simulink model "Comparison_to_Nest"  (R2020b)
settings: Solver=VariableStepAuto  StartTime=0.0  StopTime=0.4  RelTol=1e-3
libraries: NeuroModelerLibrary x7
settings Model: Creator=Александра  LastModifiedBy=Александра

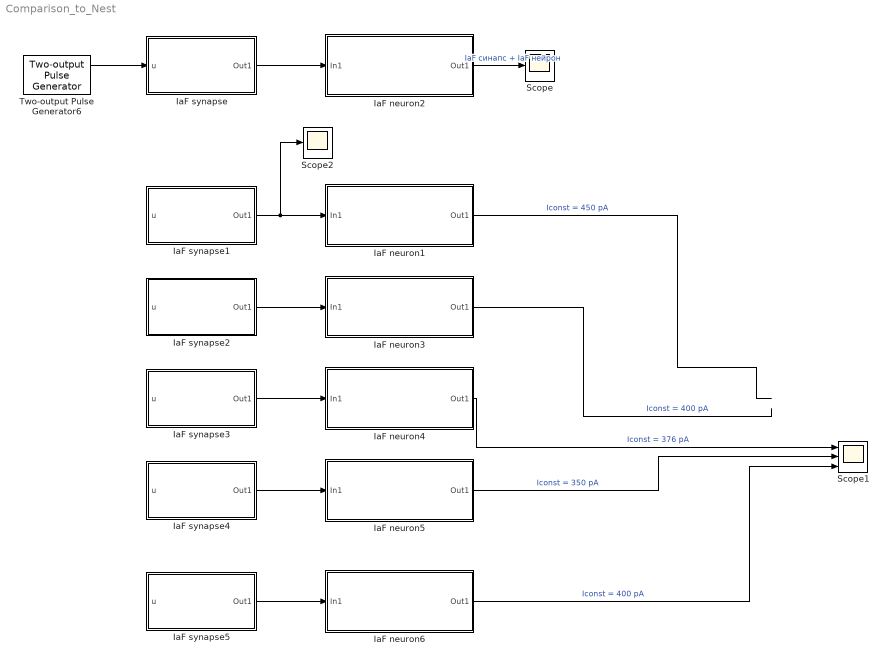
== system Comparison_to_Nest ==
  IaF neuron1 : Subsystem  mask{tau_m=0.010, Cm=250e-12, I_const=450e-12, E_L=-0.070, V_reset=-0.070, V_th=-0.055}
      mask prompts: tau_m "Membrane time constatnt"; Cm "Membrane capacity"; I_const "Constant input current"; E_L "Resting membrane potential"; V_reset "Reset membrane potential"; V_th "Threshold potential"
  IaF neuron2 : Subsystem  mask{tau_m=0.01, Cm=250e-12, I_const=0, E_L=-0.070, V_reset=-0.10, V_th=-0.055}
      mask prompts: tau_m "Membrane time constatnt"; Cm "Membrane capacity"; I_const "Constant input current"; E_L "Resting membrane potential"; V_reset "Reset membrane potential"; V_th "Threshold potential"
  IaF neuron3 : Subsystem  mask{tau_m=0.010, Cm=250e-12, I_const=400e-12, E_L=-0.070, V_reset=-0.070, V_th=-0.055}
      mask prompts: tau_m "Membrane time constatnt"; Cm "Membrane capacity"; I_const "Constant input current"; E_L "Resting membrane potential"; V_reset "Reset membrane potential"; V_th "Threshold potential"
  IaF neuron4 : Subsystem  mask{tau_m=0.010, Cm=250e-12, I_const=376e-12, E_L=-0.070, V_reset=-0.070, V_th=-0.055}
      mask prompts: tau_m "Membrane time constatnt"; Cm "Membrane capacity"; I_const "Constant input current"; E_L "Resting membrane potential"; V_reset "Reset membrane potential"; V_th "Threshold potential"
  IaF neuron5 : Subsystem  mask{tau_m=0.010, Cm=250e-12, I_const=350e-12, E_L=-0.070, V_reset=-0.070, V_th=-0.055}
      mask prompts: tau_m "Membrane time constatnt"; Cm "Membrane capacity"; I_const "Constant input current"; E_L "Resting membrane potential"; V_reset "Reset membrane potential"; V_th "Threshold potential"
  IaF neuron6 : Subsystem  mask{tau_m=0.010, Cm=250e-12, I_const=400e-12, E_L=-0.070, V_reset=-0.070, V_th=-0.055}
      mask prompts: tau_m "Membrane time constatnt"; Cm "Membrane capacity"; I_const "Constant input current"; E_L "Resting membrane potential"; V_reset "Reset membrane potential"; V_th "Threshold potential"
  IaF synapse : Subsystem  mask{tau_syn=2e-3, I_syn=1e-8, weight=1, delay=1e-3}
      mask prompts: tau_syn "Rise time of the excitatory synaptic alpha function"; I_syn "Synaptic current amplitude"
  IaF synapse1 : Subsystem  mask{tau_syn=2e-3, I_syn=1e-8, weight=1, delay=1e-3}
      mask prompts: tau_syn "Rise time of the excitatory synaptic alpha function"; I_syn "Synaptic current amplitude"
  IaF synapse2 : Subsystem  mask{tau_syn=2e-3, I_syn=1e-8, weight=1, delay=1e-3}
      mask prompts: tau_syn "Rise time of the excitatory synaptic alpha function"; I_syn "Synaptic current amplitude"
  IaF synapse3 : Subsystem  mask{tau_syn=2e-3, I_syn=1e-8, weight=1, delay=1e-3}
      mask prompts: tau_syn "Rise time of the excitatory synaptic alpha function"; I_syn "Synaptic current amplitude"
  IaF synapse4 : Subsystem  mask{tau_syn=2e-3, I_syn=1e-8, weight=1, delay=1e-3}
      mask prompts: tau_syn "Rise time of the excitatory synaptic alpha function"; I_syn "Synaptic current amplitude"
  IaF synapse5 : Subsystem  mask{tau_syn=2e-3, I_syn=1e-8, weight=1, delay=1e-3}
      mask prompts: tau_syn "Rise time of the excitatory synaptic alpha function"; I_syn "Synaptic current amplitude"
  Scope : Scope
  Scope1 : Scope  NumInputPorts=3
  Scope2 : Scope
  Two-output Pulse Generator6 : NeuroModelerLibrary/Support/Two-output Pulse Generator  A=1  P1=200  P2=200  PW=1  ST=0.001  OOn1=0.1  OOff1=1.0  OOn2=0.1  OOff2=0.2
  wires:
  Two-output Pulse Generator6/1 -> IaF synapse/1(u)
  IaF synapse/1(Out1) -> IaF neuron2/1(In1)
  IaF neuron2/1(Out1) -> Scope/1  "IaF синапс + IaF нейрон"
  IaF neuron1/1(Out1) -> ?  "Iconst = 450 pA"
  IaF synapse1/1(Out1) -> Scope2/1, IaF neuron1/1(In1)
  IaF neuron3/1(Out1) -> ?  "Iconst = 400 pA"
  IaF synapse2/1(Out1) -> IaF neuron3/1(In1)
  IaF neuron4/1(Out1) -> Scope1/1  "Iconst = 376 pA"
  IaF synapse3/1(Out1) -> IaF neuron4/1(In1)
  IaF synapse4/1(Out1) -> IaF neuron5/1(In1)
  IaF synapse5/1(Out1) -> IaF neuron6/1(In1)
  IaF neuron5/1(Out1) -> Scope1/2  "Iconst = 350 pA"
  IaF neuron6/1(Out1) -> Scope1/3  "Iconst = 400 pA"

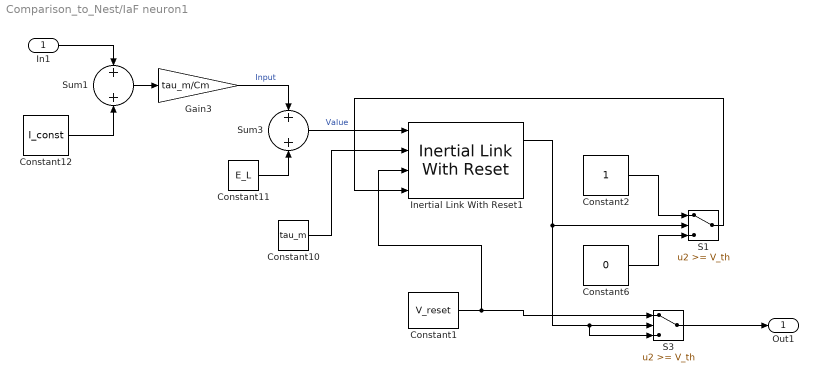
== system Comparison_to_Nest/IaF neuron1 ==
  In1 : Inport
  Constant1 : Constant  Value=V_reset
  Constant10 : Constant  Value=tau_m
  Constant11 : Constant  Value=E_L
  Constant12 : Constant  Value=I_const
  Constant2 : Constant
  Constant6 : Constant  Value=0
  Gain3 : Gain  Gain=tau_m/Cm
  Inertial Link With Reset1 : NeuroModelerLibrary/Support/Inertial Link With Reset  SystemSampleTime=-1  VariantActivationTime=update diagram  Latency=0  AutoFrameSizeCalculation=off
  S1 : Switch  Threshold=V_th  SaturateOnIntegerOverflow=on  InputSameDT=on
  S3 : Switch  Threshold=V_th  SaturateOnIntegerOverflow=on  InputSameDT=on
  Sum1 : Sum
  Sum3 : Sum
  Out1 : Outport
  wires:
  Constant11/1 -> Sum3/2
  Constant10/1 -> Inertial Link With Reset1/2
  In1/1 -> Sum1/1
  Sum1/1 -> Gain3/1
  Constant12/1 -> Sum1/2
  Constant2/1 -> S1/1
  Constant6/1 -> S1/3
  Sum3/1 -> Inertial Link With Reset1/1  "Value"
  Inertial Link With Reset1/1 -> S1/2, S3/3, S3/2
  Constant1/1 -> Inertial Link With Reset1/3, S3/1
  S1/1 -> Inertial Link With Reset1/4
  S3/1 -> Out1/1
  Gain3/1 -> Sum3/1  "Input"

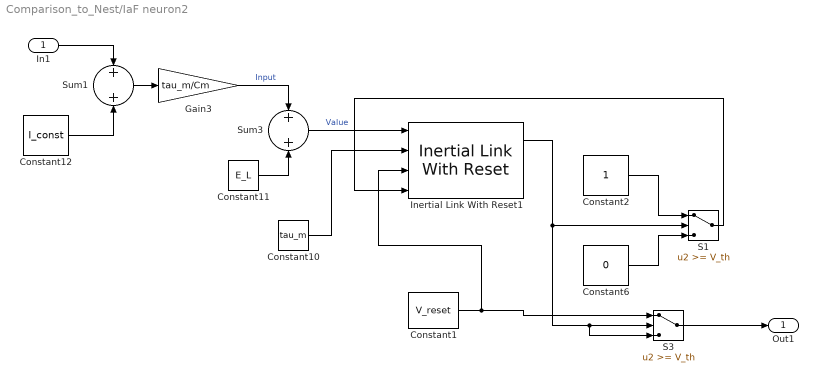
== system Comparison_to_Nest/IaF neuron2 ==
  In1 : Inport
  Constant1 : Constant  Value=V_reset
  Constant10 : Constant  Value=tau_m
  Constant11 : Constant  Value=E_L
  Constant12 : Constant  Value=I_const
  Constant2 : Constant
  Constant6 : Constant  Value=0
  Gain3 : Gain  Gain=tau_m/Cm
  Inertial Link With Reset1 : NeuroModelerLibrary/Support/Inertial Link With Reset  SystemSampleTime=-1  VariantActivationTime=update diagram  Latency=0  AutoFrameSizeCalculation=off
  S1 : Switch  Threshold=V_th  SaturateOnIntegerOverflow=on  InputSameDT=on
  S3 : Switch  Threshold=V_th  SaturateOnIntegerOverflow=on  InputSameDT=on
  Sum1 : Sum
  Sum3 : Sum
  Out1 : Outport
  wires:
  Constant11/1 -> Sum3/2
  Constant10/1 -> Inertial Link With Reset1/2
  In1/1 -> Sum1/1
  Sum1/1 -> Gain3/1
  Constant12/1 -> Sum1/2
  Constant2/1 -> S1/1
  Constant6/1 -> S1/3
  Sum3/1 -> Inertial Link With Reset1/1  "Value"
  Inertial Link With Reset1/1 -> S1/2, S3/3, S3/2
  Constant1/1 -> Inertial Link With Reset1/3, S3/1
  S1/1 -> Inertial Link With Reset1/4
  S3/1 -> Out1/1
  Gain3/1 -> Sum3/1  "Input"

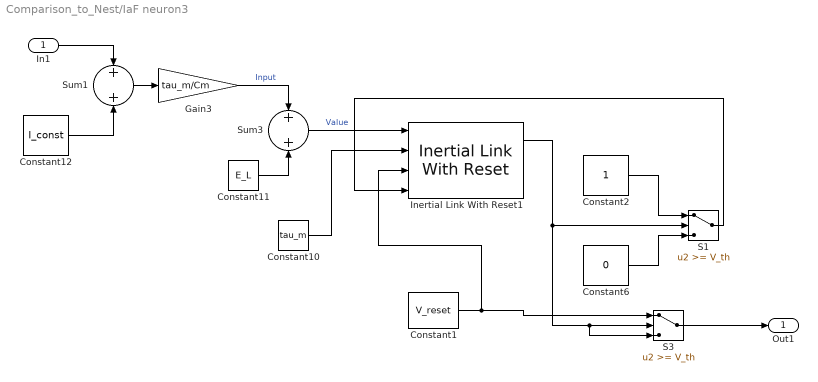
== system Comparison_to_Nest/IaF neuron3 ==
  In1 : Inport
  Constant1 : Constant  Value=V_reset
  Constant10 : Constant  Value=tau_m
  Constant11 : Constant  Value=E_L
  Constant12 : Constant  Value=I_const
  Constant2 : Constant
  Constant6 : Constant  Value=0
  Gain3 : Gain  Gain=tau_m/Cm
  Inertial Link With Reset1 : NeuroModelerLibrary/Support/Inertial Link With Reset  SystemSampleTime=-1  VariantActivationTime=update diagram  Latency=0  AutoFrameSizeCalculation=off
  S1 : Switch  Threshold=V_th  SaturateOnIntegerOverflow=on  InputSameDT=on
  S3 : Switch  Threshold=V_th  SaturateOnIntegerOverflow=on  InputSameDT=on
  Sum1 : Sum
  Sum3 : Sum
  Out1 : Outport
  wires:
  Constant11/1 -> Sum3/2
  Constant10/1 -> Inertial Link With Reset1/2
  In1/1 -> Sum1/1
  Sum1/1 -> Gain3/1
  Constant12/1 -> Sum1/2
  Constant2/1 -> S1/1
  Constant6/1 -> S1/3
  Sum3/1 -> Inertial Link With Reset1/1  "Value"
  Inertial Link With Reset1/1 -> S1/2, S3/3, S3/2
  Constant1/1 -> Inertial Link With Reset1/3, S3/1
  S1/1 -> Inertial Link With Reset1/4
  S3/1 -> Out1/1
  Gain3/1 -> Sum3/1  "Input"

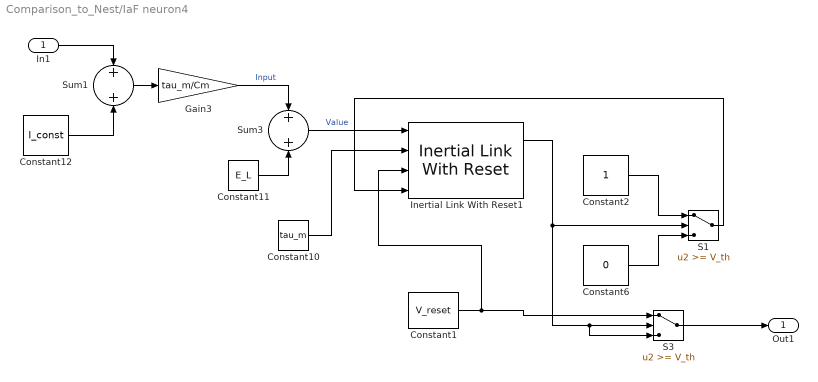
== system Comparison_to_Nest/IaF neuron4 ==
  In1 : Inport
  Constant1 : Constant  Value=V_reset
  Constant10 : Constant  Value=tau_m
  Constant11 : Constant  Value=E_L
  Constant12 : Constant  Value=I_const
  Constant2 : Constant
  Constant6 : Constant  Value=0
  Gain3 : Gain  Gain=tau_m/Cm
  Inertial Link With Reset1 : NeuroModelerLibrary/Support/Inertial Link With Reset  SystemSampleTime=-1  VariantActivationTime=update diagram  Latency=0  AutoFrameSizeCalculation=off
  S1 : Switch  Threshold=V_th  SaturateOnIntegerOverflow=on  InputSameDT=on
  S3 : Switch  Threshold=V_th  SaturateOnIntegerOverflow=on  InputSameDT=on
  Sum1 : Sum
  Sum3 : Sum
  Out1 : Outport
  wires:
  Constant11/1 -> Sum3/2
  Constant10/1 -> Inertial Link With Reset1/2
  In1/1 -> Sum1/1
  Sum1/1 -> Gain3/1
  Constant12/1 -> Sum1/2
  Constant2/1 -> S1/1
  Constant6/1 -> S1/3
  Sum3/1 -> Inertial Link With Reset1/1  "Value"
  Inertial Link With Reset1/1 -> S1/2, S3/3, S3/2
  Constant1/1 -> Inertial Link With Reset1/3, S3/1
  S1/1 -> Inertial Link With Reset1/4
  S3/1 -> Out1/1
  Gain3/1 -> Sum3/1  "Input"

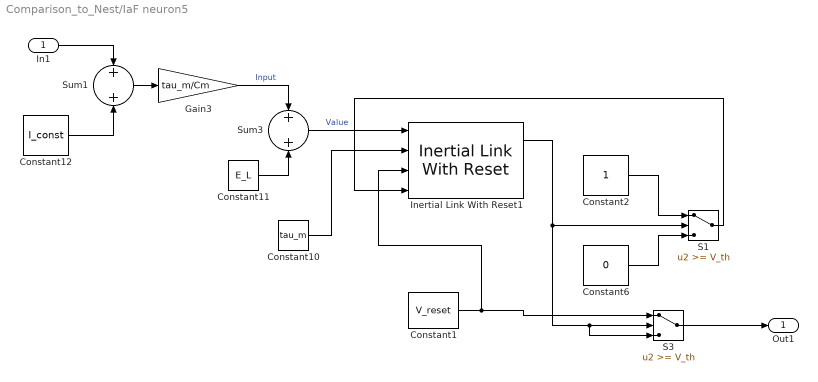
== system Comparison_to_Nest/IaF neuron5 ==
  In1 : Inport
  Constant1 : Constant  Value=V_reset
  Constant10 : Constant  Value=tau_m
  Constant11 : Constant  Value=E_L
  Constant12 : Constant  Value=I_const
  Constant2 : Constant
  Constant6 : Constant  Value=0
  Gain3 : Gain  Gain=tau_m/Cm
  Inertial Link With Reset1 : NeuroModelerLibrary/Support/Inertial Link With Reset  SystemSampleTime=-1  VariantActivationTime=update diagram  Latency=0  AutoFrameSizeCalculation=off
  S1 : Switch  Threshold=V_th  SaturateOnIntegerOverflow=on  InputSameDT=on
  S3 : Switch  Threshold=V_th  SaturateOnIntegerOverflow=on  InputSameDT=on
  Sum1 : Sum
  Sum3 : Sum
  Out1 : Outport
  wires:
  Constant11/1 -> Sum3/2
  Constant10/1 -> Inertial Link With Reset1/2
  In1/1 -> Sum1/1
  Sum1/1 -> Gain3/1
  Constant12/1 -> Sum1/2
  Constant2/1 -> S1/1
  Constant6/1 -> S1/3
  Sum3/1 -> Inertial Link With Reset1/1  "Value"
  Inertial Link With Reset1/1 -> S1/2, S3/3, S3/2
  Constant1/1 -> Inertial Link With Reset1/3, S3/1
  S1/1 -> Inertial Link With Reset1/4
  S3/1 -> Out1/1
  Gain3/1 -> Sum3/1  "Input"

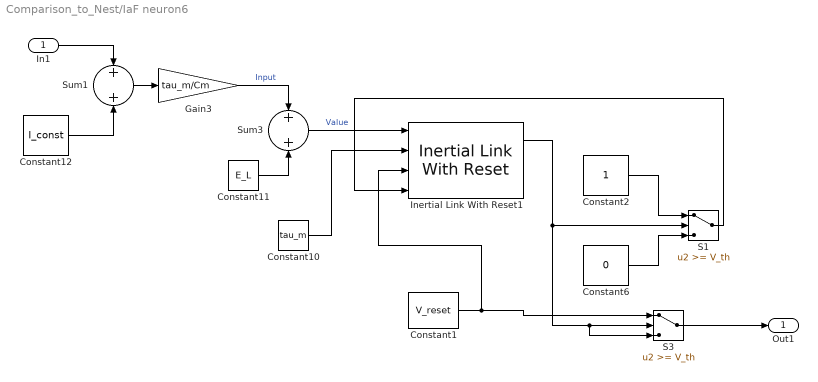
== system Comparison_to_Nest/IaF neuron6 ==
  In1 : Inport
  Constant1 : Constant  Value=V_reset
  Constant10 : Constant  Value=tau_m
  Constant11 : Constant  Value=E_L
  Constant12 : Constant  Value=I_const
  Constant2 : Constant
  Constant6 : Constant  Value=0
  Gain3 : Gain  Gain=tau_m/Cm
  Inertial Link With Reset1 : NeuroModelerLibrary/Support/Inertial Link With Reset  SystemSampleTime=-1  VariantActivationTime=update diagram  Latency=0  AutoFrameSizeCalculation=off
  S1 : Switch  Threshold=V_th  SaturateOnIntegerOverflow=on  InputSameDT=on
  S3 : Switch  Threshold=V_th  SaturateOnIntegerOverflow=on  InputSameDT=on
  Sum1 : Sum
  Sum3 : Sum
  Out1 : Outport
  wires:
  Constant11/1 -> Sum3/2
  Constant10/1 -> Inertial Link With Reset1/2
  In1/1 -> Sum1/1
  Sum1/1 -> Gain3/1
  Constant12/1 -> Sum1/2
  Constant2/1 -> S1/1
  Constant6/1 -> S1/3
  Sum3/1 -> Inertial Link With Reset1/1  "Value"
  Inertial Link With Reset1/1 -> S1/2, S3/3, S3/2
  Constant1/1 -> Inertial Link With Reset1/3, S3/1
  S1/1 -> Inertial Link With Reset1/4
  S3/1 -> Out1/1
  Gain3/1 -> Sum3/1  "Input"

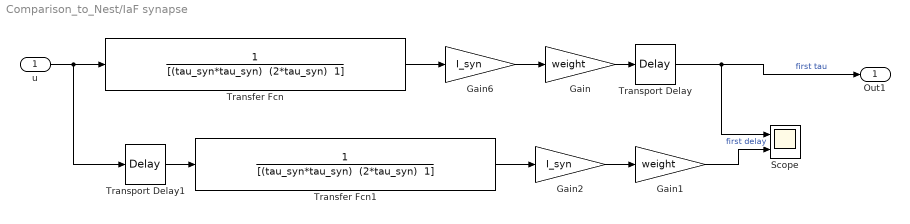
== system Comparison_to_Nest/IaF synapse ==
  u : Inport
  Gain : Gain  Gain=weight
  Gain1 : Gain  Gain=weight
  Gain2 : Gain  Gain=I_syn
  Gain6 : Gain  Gain=I_syn
  Scope : Scope  NumInputPorts=2
  Transfer Fcn : TransferFcn  Denominator="[(tau_syn*tau_syn)  (2*tau_syn)  1]"
  Transfer Fcn1 : TransferFcn  Denominator="[(tau_syn*tau_syn)  (2*tau_syn)  1]"
  Transport Delay : TransportDelay  DelayTime=delay
  Transport Delay1 : TransportDelay  DelayTime=delay
  Out1 : Outport
  wires:
  Transport Delay/1 -> Scope/1, Out1/1  "first tau"
  Gain/1 -> Transport Delay/1
  Gain6/1 -> Gain/1
  Transfer Fcn/1 -> Gain6/1
  u/1 -> Transport Delay1/1, Transfer Fcn/1
  Transfer Fcn1/1 -> Gain2/1
  Gain2/1 -> Gain1/1
  Transport Delay1/1 -> Transfer Fcn1/1
  Gain1/1 -> Scope/2  "first delay"

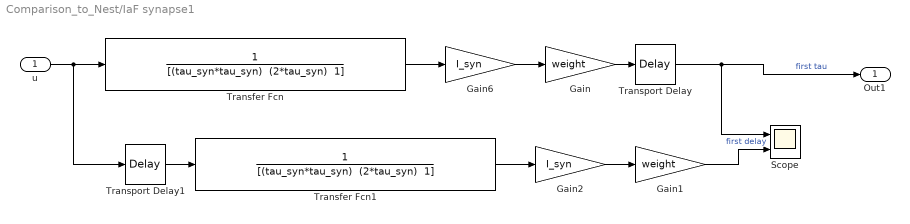
== system Comparison_to_Nest/IaF synapse1 ==
  u : Inport
  Gain : Gain  Gain=weight
  Gain1 : Gain  Gain=weight
  Gain2 : Gain  Gain=I_syn
  Gain6 : Gain  Gain=I_syn
  Scope : Scope  NumInputPorts=2
  Transfer Fcn : TransferFcn  Denominator="[(tau_syn*tau_syn)  (2*tau_syn)  1]"
  Transfer Fcn1 : TransferFcn  Denominator="[(tau_syn*tau_syn)  (2*tau_syn)  1]"
  Transport Delay : TransportDelay  DelayTime=delay
  Transport Delay1 : TransportDelay  DelayTime=delay
  Out1 : Outport
  wires:
  Transport Delay/1 -> Scope/1, Out1/1  "first tau"
  Gain/1 -> Transport Delay/1
  Gain6/1 -> Gain/1
  Transfer Fcn/1 -> Gain6/1
  u/1 -> Transport Delay1/1, Transfer Fcn/1
  Transfer Fcn1/1 -> Gain2/1
  Gain2/1 -> Gain1/1
  Transport Delay1/1 -> Transfer Fcn1/1
  Gain1/1 -> Scope/2  "first delay"

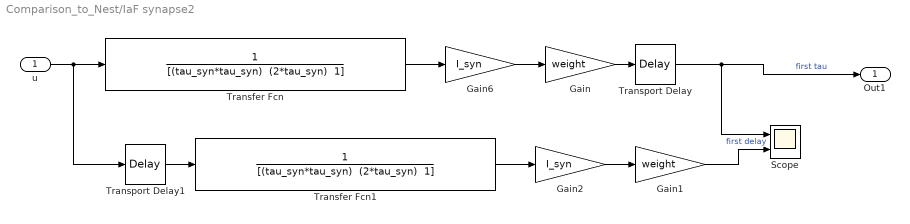
== system Comparison_to_Nest/IaF synapse2 ==
  u : Inport
  Gain : Gain  Gain=weight
  Gain1 : Gain  Gain=weight
  Gain2 : Gain  Gain=I_syn
  Gain6 : Gain  Gain=I_syn
  Scope : Scope  NumInputPorts=2
  Transfer Fcn : TransferFcn  Denominator="[(tau_syn*tau_syn)  (2*tau_syn)  1]"
  Transfer Fcn1 : TransferFcn  Denominator="[(tau_syn*tau_syn)  (2*tau_syn)  1]"
  Transport Delay : TransportDelay  DelayTime=delay
  Transport Delay1 : TransportDelay  DelayTime=delay
  Out1 : Outport
  wires:
  Transport Delay/1 -> Scope/1, Out1/1  "first tau"
  Gain/1 -> Transport Delay/1
  Gain6/1 -> Gain/1
  Transfer Fcn/1 -> Gain6/1
  u/1 -> Transport Delay1/1, Transfer Fcn/1
  Transfer Fcn1/1 -> Gain2/1
  Gain2/1 -> Gain1/1
  Transport Delay1/1 -> Transfer Fcn1/1
  Gain1/1 -> Scope/2  "first delay"

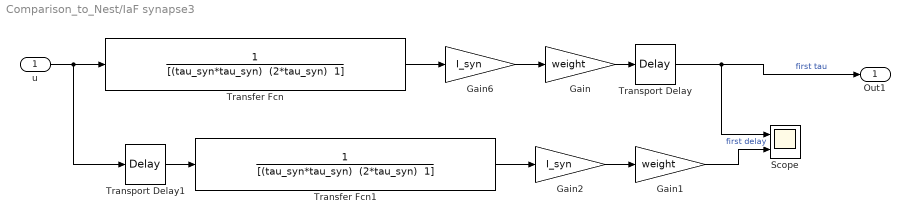
== system Comparison_to_Nest/IaF synapse3 ==
  u : Inport
  Gain : Gain  Gain=weight
  Gain1 : Gain  Gain=weight
  Gain2 : Gain  Gain=I_syn
  Gain6 : Gain  Gain=I_syn
  Scope : Scope  NumInputPorts=2
  Transfer Fcn : TransferFcn  Denominator="[(tau_syn*tau_syn)  (2*tau_syn)  1]"
  Transfer Fcn1 : TransferFcn  Denominator="[(tau_syn*tau_syn)  (2*tau_syn)  1]"
  Transport Delay : TransportDelay  DelayTime=delay
  Transport Delay1 : TransportDelay  DelayTime=delay
  Out1 : Outport
  wires:
  Transport Delay/1 -> Scope/1, Out1/1  "first tau"
  Gain/1 -> Transport Delay/1
  Gain6/1 -> Gain/1
  Transfer Fcn/1 -> Gain6/1
  u/1 -> Transport Delay1/1, Transfer Fcn/1
  Transfer Fcn1/1 -> Gain2/1
  Gain2/1 -> Gain1/1
  Transport Delay1/1 -> Transfer Fcn1/1
  Gain1/1 -> Scope/2  "first delay"

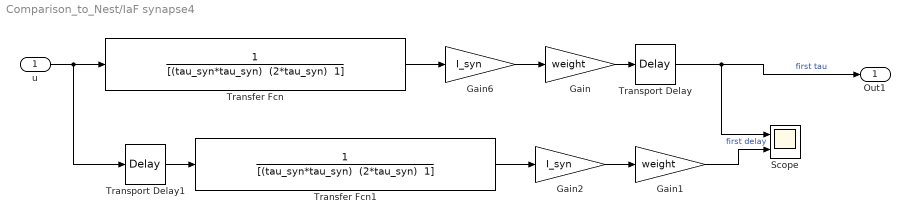
== system Comparison_to_Nest/IaF synapse4 ==
  u : Inport
  Gain : Gain  Gain=weight
  Gain1 : Gain  Gain=weight
  Gain2 : Gain  Gain=I_syn
  Gain6 : Gain  Gain=I_syn
  Scope : Scope  NumInputPorts=2
  Transfer Fcn : TransferFcn  Denominator="[(tau_syn*tau_syn)  (2*tau_syn)  1]"
  Transfer Fcn1 : TransferFcn  Denominator="[(tau_syn*tau_syn)  (2*tau_syn)  1]"
  Transport Delay : TransportDelay  DelayTime=delay
  Transport Delay1 : TransportDelay  DelayTime=delay
  Out1 : Outport
  wires:
  Transport Delay/1 -> Scope/1, Out1/1  "first tau"
  Gain/1 -> Transport Delay/1
  Gain6/1 -> Gain/1
  Transfer Fcn/1 -> Gain6/1
  u/1 -> Transport Delay1/1, Transfer Fcn/1
  Transfer Fcn1/1 -> Gain2/1
  Gain2/1 -> Gain1/1
  Transport Delay1/1 -> Transfer Fcn1/1
  Gain1/1 -> Scope/2  "first delay"

== system Comparison_to_Nest/IaF synapse5 ==
  u : Inport
  Gain : Gain  Gain=weight
  Gain1 : Gain  Gain=weight
  Gain2 : Gain  Gain=I_syn
  Gain6 : Gain  Gain=I_syn
  Scope : Scope  NumInputPorts=2
  Transfer Fcn : TransferFcn  Denominator="[(tau_syn*tau_syn)  (2*tau_syn)  1]"
  Transfer Fcn1 : TransferFcn  Denominator="[(tau_syn*tau_syn)  (2*tau_syn)  1]"
  Transport Delay : TransportDelay  DelayTime=delay
  Transport Delay1 : TransportDelay  DelayTime=delay
  Out1 : Outport
  wires:
  Transport Delay/1 -> Scope/1, Out1/1  "first tau"
  Gain/1 -> Transport Delay/1
  Gain6/1 -> Gain/1
  Transfer Fcn/1 -> Gain6/1
  u/1 -> Transport Delay1/1, Transfer Fcn/1
  Transfer Fcn1/1 -> Gain2/1
  Gain2/1 -> Gain1/1
  Transport Delay1/1 -> Transfer Fcn1/1
  Gain1/1 -> Scope/2  "first delay"
